simulink model "sensorFusion"  (R2016b)
settings: configuration reference "Run_on_Hardware_Configuration2" (kept outside this file)
values from neighbouring files (symbols this model uses):
  aMean = -0.038579232696484993 0.015125405229726172 0.985264268406069    [quadCopterDD.sldd]
  aVar = 5.1253776232526919E-6 4.2277820138033229E-6 1.1915659975536502E-5    [quadCopterDD.sldd]
  gMean = -0.0070511589569554516 0.0038285549128950222 0.011166026028447077    [quadCopterDD.sldd]
  mMean = 47.735714991803668 -38.636009827303312 87.517185038334446    [quadCopterDD.sldd]
  mVar = 39.430756512955334 40.815922310000467 35.444708601605633    [quadCopterDD.sldd]
libraries: simulink x1, embdlinuxlib x1
settings Model: DataDictionary=quadCopterDD.sldd  SimulationMode=external  Creator=nikol  LastModifiedBy=nikol
settings ConfigSetRef: DDName=quadCopterDD.sldd

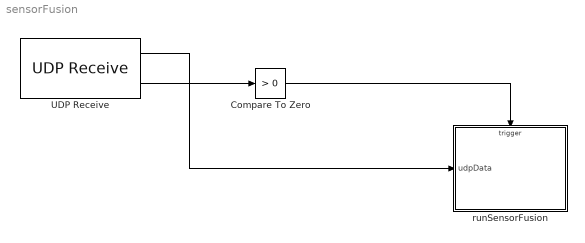
== system sensorFusion ==
  Compare To Zero : simulink/Logic and Bit Operations/Compare To Zero  relop=>  OutDataTypeStr=boolean
  UDP Receive : embdlinuxlib/UDP Receive  localURL='0.0.0.0'  localPort=25000  remoteURL='0.0.0.0'  remotePort=-1  recvBufferSize=8192  signalDatatype=single  dims=32  isVarSize=off  showBlockingTime=off  blockingTime=0  sampletime=1/1000  blockPlatform=Raspberry Pi
  runSensorFusion : Subsystem  TreatAsAtomicUnit=on
  wires:
  UDP Receive/1 -> runSensorFusion/1(udpData)
  Compare To Zero/1 -> runSensorFusion/Trigger
  UDP Receive/2 -> Compare To Zero/1

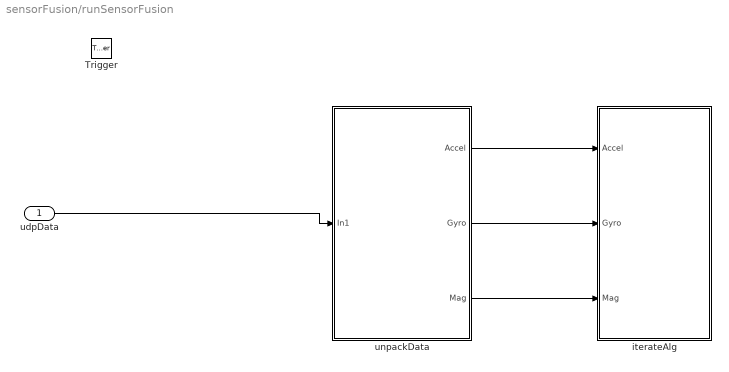
== system sensorFusion/runSensorFusion ==
  udpData : Inport
  Trigger : TriggerPort  VariantControl=Variant  PortDimensions=1
  iterateAlg : Subsystem  TreatAsAtomicUnit=on
  unpackData : Subsystem
  wires:
  unpackData/3(Mag) -> iterateAlg/3(Mag)
  unpackData/2(Gyro) -> iterateAlg/2(Gyro)
  unpackData/1(Accel) -> iterateAlg/1(Accel)
  udpData/1 -> unpackData/1(In1)

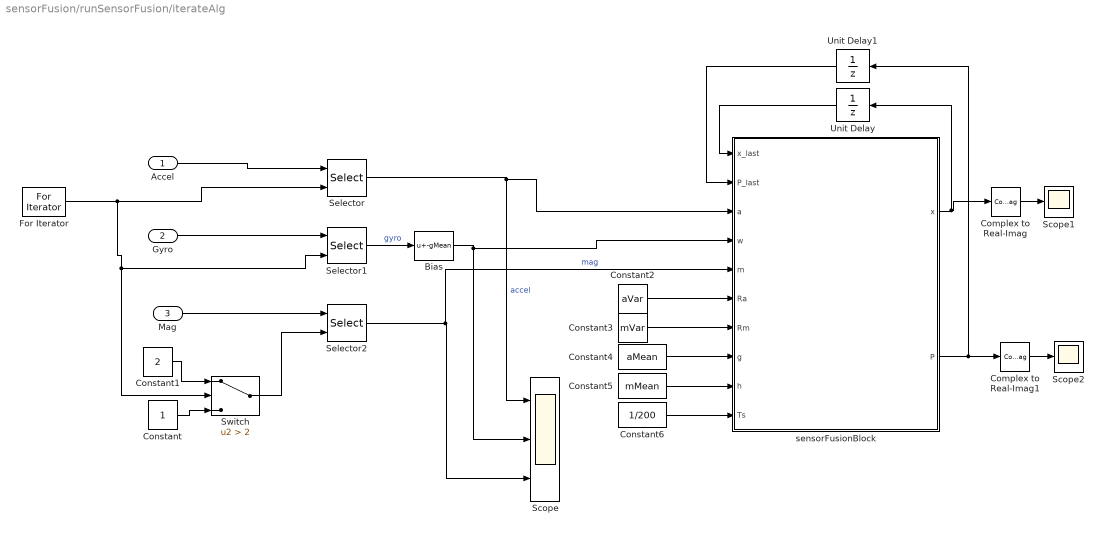
== system sensorFusion/runSensorFusion/iterateAlg ==
  Accel : Inport
  Gyro : Inport  Port=2
  Mag : Inport  Port=3
  Bias : Bias  Bias=-gMean
  Complex to Real-Imag : ComplexToRealImag  Output=Real
  Complex to Real-Imag1 : ComplexToRealImag  Output=Real
  Constant : Constant  OutDataTypeStr=int32
  Constant1 : Constant  Value=2  OutDataTypeStr=int32
  Constant2 : Constant  Value=aVar
  Constant3 : Constant  Value=mVar
  Constant4 : Constant  Value=aMean
  Constant5 : Constant  Value=mMean
  Constant6 : Constant  Value=1/200
  For Iterator : ForIterator  IterationLimit=4
  Scope : Scope  NumInputPorts=3
  Scope1 : Scope
  Scope2 : Scope
  Selector : Selector  NumberOfDimensions=2  InputPortWidth=3  IndexOptions=Index vector (dialog),Index vector (port)  Indices=[1 2 3],1  OutputSizes=1,1
  Selector1 : Selector  NumberOfDimensions=2  InputPortWidth=3  IndexOptions=Index vector (dialog),Index vector (port)  Indices=[1 2 3],1  OutputSizes=1,1
  Selector2 : Selector  NumberOfDimensions=2  InputPortWidth=3  IndexOptions=Index vector (dialog),Index vector (port)  Indices=[1 2 3],1  OutputSizes=1,1
  Switch : Switch  Criteria=u2 > Threshold  Threshold=2
  Unit Delay : UnitDelay  InitialCondition=single([0 0 0 1])  SampleTime=-1
  Unit Delay1 : UnitDelay  InitialCondition=single(eye(4))  SampleTime=-1
  sensorFusionBlock : MATLAB Function  TreatAsAtomicUnit=on
  wires:
  For Iterator/1 -> Switch/2, Selector1/2, Selector/2
  Accel/1 -> Selector/1
  Gyro/1 -> Selector1/1
  Constant/1 -> Switch/3
  Constant1/1 -> Switch/1
  Switch/1 -> Selector2/2
  Mag/1 -> Selector2/1
  Selector/1 -> sensorFusionBlock/3(a), Scope/1  "accel"
  Selector1/1 -> Bias/1  "gyro"
  Selector2/1 -> sensorFusionBlock/5(m), Scope/3  "mag"
  Bias/1 -> sensorFusionBlock/4(w), Scope/2
  sensorFusionBlock/1(x) -> Complex to Real-Imag/1, Unit Delay/1
  Unit Delay/1 -> sensorFusionBlock/1(x_last)
  sensorFusionBlock/2(P) -> Complex to Real-Imag1/1, Unit Delay1/1
  Unit Delay1/1 -> sensorFusionBlock/2(P_last)
  Constant2/1 -> sensorFusionBlock/6(Ra)
  Constant3/1 -> sensorFusionBlock/7(Rm)
  Constant4/1 -> sensorFusionBlock/8(g)
  Constant5/1 -> sensorFusionBlock/9(h)
  Constant6/1 -> sensorFusionBlock/10(Ts)
  Complex to Real-Imag/1 -> Scope1/1
  Complex to Real-Imag1/1 -> Scope2/1

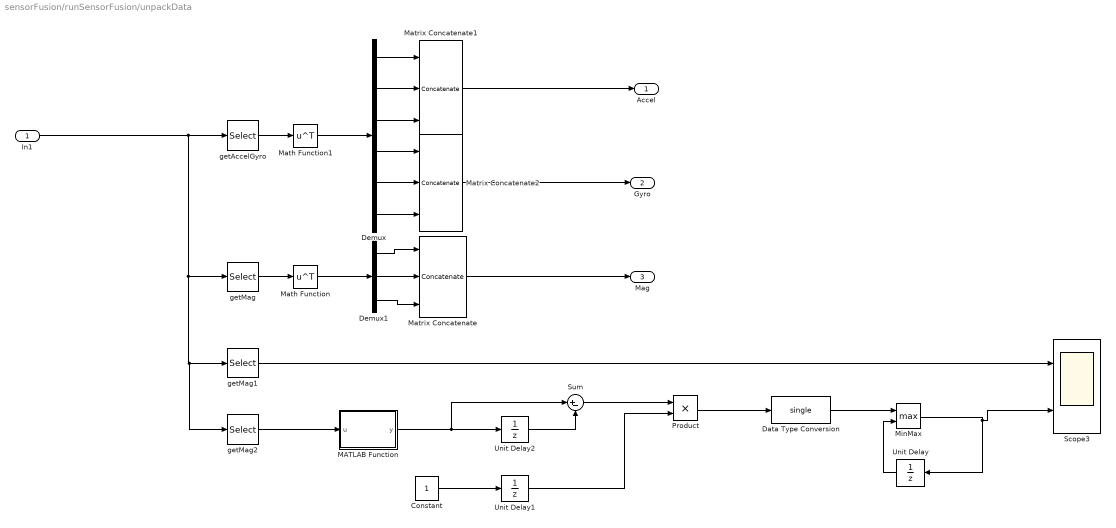
== system sensorFusion/runSensorFusion/unpackData ==
  In1 : Inport
  Constant : Constant  OutDataTypeStr=uint32
  Data Type Conversion : DataTypeConversion  OutDataTypeStr=single
  Demux : Demux  Outputs=6
  Demux1 : Demux  Outputs=3
  MATLAB Function : MATLAB Function  TreatAsAtomicUnit=on
  Math Function : Math  Operator=transpose  SaturateOnIntegerOverflow=on
  Math Function1 : Math  Operator=transpose  SaturateOnIntegerOverflow=on
  Matrix Concatenate : Concatenate  NumInputs=3  Mode=Multidimensional array
  Matrix Concatenate1 : Concatenate  NumInputs=3  Mode=Multidimensional array
  Matrix Concatenate2 : Concatenate  NumInputs=3  Mode=Multidimensional array
  MinMax : MinMax  Function=max  Inputs=2
  Product : Product
  Scope3 : Scope  NumInputPorts=2
  Sum : Sum  Inputs=|+-
  Unit Delay : UnitDelay  SampleTime=-1
  Unit Delay1 : UnitDelay  SampleTime=-1
  Unit Delay2 : UnitDelay  SampleTime=-1
  getAccelGyro : Selector  InputPortWidth=32  IndexOptions=Index vector (dialog)  Indices=1:24  OutputSizes=1
  getMag : Selector  InputPortWidth=32  IndexOptions=Index vector (dialog)  Indices=25:30  OutputSizes=1
  getMag1 : Selector  InputPortWidth=32  IndexOptions=Index vector (dialog)  Indices=31  OutputSizes=1
  getMag2 : Selector  InputPortWidth=32  IndexOptions=Index vector (dialog)  Indices=32  OutputSizes=1
  Accel : Outport
  Gyro : Outport  Port=2
  Mag : Outport  Port=3
  wires:
  Matrix Concatenate1/1 -> Accel/1
  Matrix Concatenate/1 -> Mag/1
  Matrix Concatenate2/1 -> Gyro/1
  Demux/6 -> Matrix Concatenate2/3
  getAccelGyro/1 -> Math Function1/1
  Math Function1/1 -> Demux/1
  Demux/5 -> Matrix Concatenate2/2
  Demux/4 -> Matrix Concatenate2/1
  Demux/1 -> Matrix Concatenate1/1
  Demux/3 -> Matrix Concatenate1/3
  Demux/2 -> Matrix Concatenate1/2
  Demux1/3 -> Matrix Concatenate/3
  Demux1/1 -> Matrix Concatenate/1
  Demux1/2 -> Matrix Concatenate/2
  getMag/1 -> Math Function/1
  In1/1 -> getAccelGyro/1, getMag2/1, getMag1/1, getMag/1
  Math Function/1 -> Demux1/1
  getMag1/1 -> Scope3/1
  getMag2/1 -> MATLAB Function/1(u)
  MATLAB Function/1(y) -> Sum/1, Unit Delay2/1
  Sum/1 -> Product/1
  Data Type Conversion/1 -> MinMax/1
  Unit Delay2/1 -> Sum/2
  Constant/1 -> Unit Delay1/1
  Unit Delay1/1 -> Product/2
  Product/1 -> Data Type Conversion/1
  MinMax/1 -> Scope3/2, Unit Delay/1
  Unit Delay/1 -> MinMax/2

== matlab function sensorFusion/runSensorFusion/unpackData/MATLAB Function ==
  data: u input; y output size=1
function y = fcn(u)

y = typecast(u,'uint32');

== matlab function sensorFusion/runSensorFusion/iterateAlg/sensorFusionBlock ==
  data: x_last input single; P_last input single; a input; w input; m input; Ra input; Rm input; g input; h input; Ts input; x output single; P output single
function [x,P]=sensorFusionEKF(x_last,P_last,a,w,m,Ra,Rm,g,h,Ts)
% Update Q
QqChi=[skew(x_last(1:3)) + x_last(4)*eye(3)
            -x_last(1:3)'];
    Q=blkdiag((Ts/2)^2*QqChi*diag(Ra)*(QqChi'));
R=single(zeros(6));
R(1,1)=Ra(1);
R(2,2)=Ra(2);
R(3,3)=Ra(3);
R(4,4)=Rm(1);
R(5,5)=Rm(2);
R(6,6)=Rm(3);

% Update Apriori Estimate and State Update Jacobian
[x_apriori,A]=stateUpdateFcn(Ts,x_last,w,true);

% Update apriori Error Covariance Estimate
P_apriori = A*P_last*A' + Q;

% Get apriori measurement and Measurement jacobian
[z_apriori,H]=measurementFcn(x_apriori,g,h,true);

% Update Kalman gain
K = (P_apriori*H') / (H*P_apriori*H' + R);

% Update aposteriori state estimate with measurement
z = [a;m];
x = x_apriori + K *(z-z_apriori);
x(1:4)=x(1:4)./norm(x(1:4));

% Update apostriori error covariance estimate
P = (eye(size(K,1)) - K*H) * P_apriori;


function [xNew,jacobian]=stateUpdateFcn(Ts,x,w,doJacobian)

wX=[0       -w(3)   w(2)
    w(3)    0       -w(1)
    -w(2)   w(1)    0];
OMEGA=complex(.5*[wX  w
          -w' 0]);

xNew=blkdiag(expm(OMEGA*Ts))*x;
xNew(1:4)=xNew(1:4)./norm(xNew(1:4));

if ~doJacobian
    return;
end

jacobian=zeros(size(xNew,1),size(xNew,1));

for i=1:length(x)
    dx=100*eps(xNew(i));
    xtemp=xNew;
    xtemp(i)=xtemp(i)+dx*1i;
    jacobian(:,i)=imag(stateUpdateFcn(Ts,xtemp,w,false))./dx;
end


function [zNew,jacobian]=measurementFcn(x,g,h,doJacobian)
b_C_n=getC(x(1:4));

zNew=blkdiag(b_C_n,b_C_n)*[g;h];

if ~doJacobian
    return;
end

jacobian=zeros(size(zNew,1),size(x,1));

for i=1:length(x)
    dx=100*eps(x(i));
    xtemp=x;
    xtemp(i)=xtemp(i)+dx*1i;
    jacobian(:,i)=imag(measurementFcn(xtemp,g,h,false))./dx;
end

function s=skew(w)
s=[0       -w(3)   w(2)
    w(3)    0       -w(1)
    -w(2)   w(1)    0];



function C=getC(q)
s=q.^2;
C=[s(1)-s(2)-s(3)+s(4)        2*(q(1)*q(2)+q(3)*q(4))    2*(q(1)*q(3)-q(2)*q(4))
   2*(q(1)*q(2)-q(3)*q(4))   -s(1)+s(2)-s(3)+s(4)        2*(q(2)*q(3)+q(4)*q(1))
   2*(q(1)*q(3)+q(2)*q(4))    2*(q(2)*q(3)-q(4)*q(1))   -s(1)-s(2)+s(3)+s(4)];
   
C=(1/sqrt(norm(q(1:3))^2+q(4)^2))*C;
